simulink model "rlwatertank"  (R2022b)
settings: Solver=FixedStepAuto  StartTime=0.0  StopTime=200.0  FixedStep=0.01  RelTol=1e-3  EnableMultiTasking=on
undefined symbols (not defined in the file): DiscIntNeverNeededParam
settings Model: DataDictionary=BusSystem.sldd  Creator=The MathWorks, Inc.  LastModifiedBy=robert
settings SolverCC: AlgebraicLoopSolver=TrustRegion
settings DataIOCC: LimitDataPoints=on  SaveOutput=off  ReturnWorkspaceOutputs=off  SignalLoggingName=logsOut
settings OptimizationCC: ExpressionDepthLimit=2147483647  InitFltsAndDblsToZero=on  LifeSpan=inf
settings DebuggingCC: SaveWithParameterizedLinksMsg=none  UnderspecifiedInitializationDetection=Classic  MergeDetectMultiDrivingBlocksExec=none  SignalResolutionControl=TryResolveAllWithWarning  MultiTaskDSMMsg=warning  FcnCallInpInsideContextMsg=warning  UnconnectedInputMsg=warning  UnconnectedOutputMsg=warning  UnconnectedLineMsg=warning  AllowSymbolicDim=off  StateNameClashWarn=warning  SFUnexpectedBacktrackingDiag=warning  SFNoUnconditionalDefaultTransitionDiag=warning  SFExecutionAtInitializationDiag=none  SFMachineParentedDataDiag=warning  ArithmeticOperatorsInVariantConditions=warning
settings HardwareCC: ProdBitPerPointer=32  ProdBitPerSizeT=32  ProdBitPerPtrDiffT=32  ProdLargestAtomicFloat=None  ProdIntDivRoundTo=Undefined  ProdEndianess=Unspecified  ProdWordSize=32  ProdHWDeviceType=Specified
settings ModelReferenceCC: EnableRefExpFcnMdlSchedulingChecks=on  PropagateSignalLabelsOutOfModel=off
settings SFSimCC: SimUseLocalCustomCode=off  CustomCodeUndefinedFunction=UseInterfaceOnly
settings RTWCC: RTWUseLocalCustomCode=off  DLArmComputeVersion=19.05
settings CodeAppCC: StateflowObjectComments=on
settings GRTTargetCC: TargetFcnLib=ansi_tfl_tmw.mat  TargetLangStandard=C89/C90 (ANSI)  CombineOutputUpdateFcns=off  GRTInterface=on
settings ConfigComp: CovMetricSettings=dw  CovSaveCumulativeToWorkspaceVar=on  CovSaveSingleToWorkspaceVar=on  CovExternalEMLEnable=off

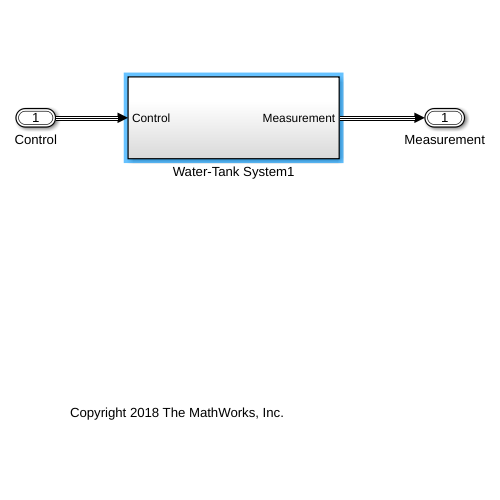
[thumbnail: Simulink's stored preview of the top-level diagram]
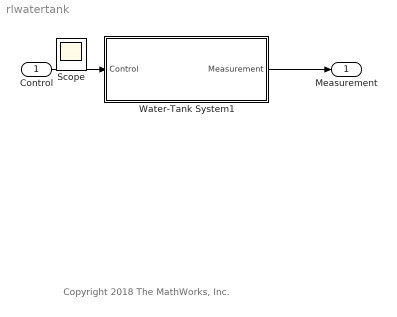
== system rlwatertank ==
  note: Copyright 2018 The MathWorks, Inc.
  Control : Inport  OutDataTypeStr=Bus: Control
  Water-Tank System1 : Subsystem
  Measurement : Outport  OutDataTypeStr=Bus: slBus3
  Scope : Scope
  wires:
  Control/1 -> Water-Tank System1/1(Control)
  Water-Tank System1/1(Measurement) -> Measurement/1

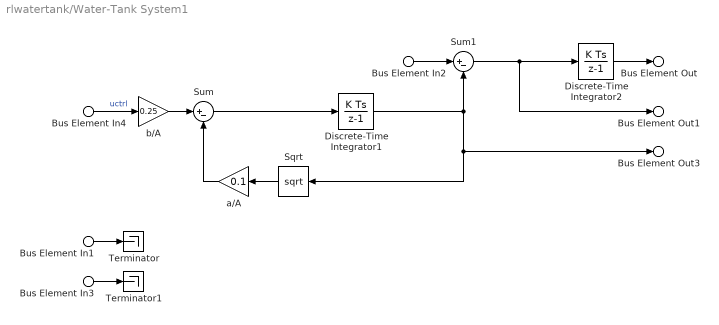
== system rlwatertank/Water-Tank System1 ==
  Bus Element In2 : Inport  PortName=Control  Element=ref
  Bus Element In4 : Inport  PortName=Control  Element=uctrl
  Bus Element In3 : Inport  PortName=Control  Element=Kidmy
  Bus Element In1 : Inport  PortName=Control  Element=Kpdmy
  Discrete-Time Integrator1 : DiscreteIntegrator  SampleTime=-1  LowerSaturationLimit=0  ICPrevOutput=DiscIntNeverNeededParam  ICPrevScaledInput=DiscIntNeverNeededParam
  Discrete-Time Integrator2 : DiscreteIntegrator  InitialCondition=3  SampleTime=-1  LowerSaturationLimit=0  ICPrevOutput=DiscIntNeverNeededParam  ICPrevScaledInput=DiscIntNeverNeededParam
  Sqrt : Sqrt  OutputSignalType=real
  Sum : Sum  Inputs=|+-  SaturateOnIntegerOverflow=on
  Sum1 : Sum  Inputs=|+-
  Terminator : Terminator
  Terminator1 : Terminator
  a/A : Gain  Gain=0.1  SaturateOnIntegerOverflow=on  OutDataTypeStr=Inherit: Same as input  ParamDataTypeStr=Inherit: Same as input
  b/A : Gain  Gain=0.25  SaturateOnIntegerOverflow=on  OutDataTypeStr=Inherit: Same as input  ParamDataTypeStr=Inherit: Same as input
  Bus Element Out : Outport  PortName=Measurement  Element=errorIntegral
  Bus Element Out1 : Outport  PortName=Measurement  Element=error
  Bus Element Out3 : Outport  PortName=Measurement  Element=height
  wires:
  a/A/1 -> Sum/2
  Sum/1 -> Discrete-Time Integrator1/1
  Sqrt/1 -> a/A/1
  Discrete-Time Integrator1/1 -> Bus Element Out3/1, Sqrt/1, Sum1/2
  Bus Element In2/1 -> Sum1/1
  Sum1/1 -> Bus Element Out1/1, Discrete-Time Integrator2/1
  Discrete-Time Integrator2/1 -> Bus Element Out/1
  b/A/1 -> Sum/1
  Bus Element In4/1 -> b/A/1  "uctrl"
  Bus Element In1/1 -> Terminator/1
  Bus Element In3/1 -> Terminator1/1
